simulink model "ALAS_NO6_SIMULINK"  (R2024a)
settings: Solver=VariableStepAuto  StartTime=0.0  StopTime=20.0  RelTol=1e-3
values from neighbouring files (symbols this model uses):
  G6_den = [t5 t4 t3 t2 t1]    [ALAS_NO6.m]    (also in ElectricalWiring.m)
  G6_num = [s4 s3 s2 s1]    [ALAS_NO6.m]    (also in ElectricalWiring.m)

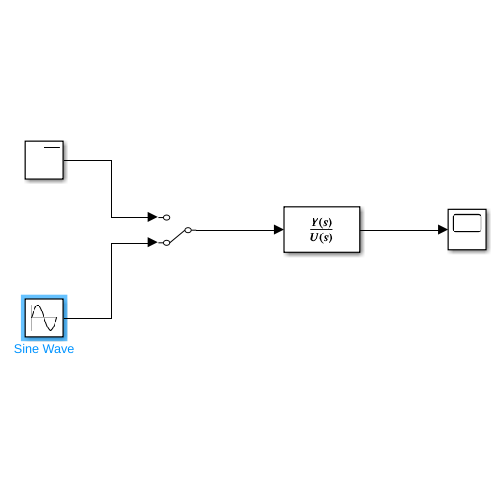
[thumbnail: Simulink's stored preview of the top-level diagram]
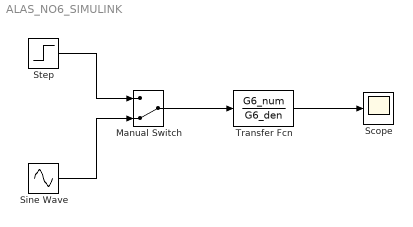
== system ALAS_NO6_SIMULINK ==
  Manual Switch : ManualSwitch  CurrentSetting=0
  Scope : Scope
  Sine Wave : Sin  SampleTime=0
  Step : Step  SampleTime=0
  Transfer Fcn : TransferFcn  Numerator=G6_num  Denominator=G6_den
  wires:
  Step/1 -> Manual Switch/1
  Sine Wave/1 -> Manual Switch/2
  Manual Switch/1 -> Transfer Fcn/1
  Transfer Fcn/1 -> Scope/1
